simulink subsystem "OFDM_modulator"  (R2022a)
settings: Solver=VariableStepAuto  StartTime=0.0  StopTime=10.0  RelTol=1e-3
values from neighbouring files (symbols this model uses):
  channelNum = fftSize / 2    (= 256)    [initSefdmModel.m]
  frameNum = dataNum + preambleNum    (= 18)    [initSefdmModel.m]
  indiciesWithCP = [issuedSize-cpLength+1:issuedSize, 1:issuedSize]    [initSefdmModel.m]
  paddingN1 = fftSize - (N1+2)    (= 256)    [initSefdmModel.m]
  symbolsPerFrame = bitsPerFrame / bitsPerSymbol    (= 4064)    [initSefdmModel.m]
libraries: dspindex x2, dspxfrm3 x1
settings Model: Creator=lsfan  LastModifiedBy=lsfan

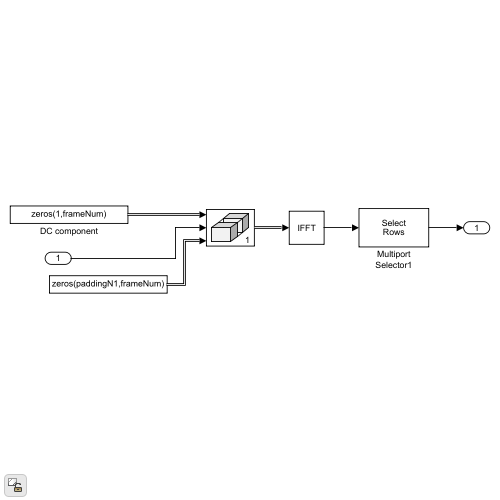
[thumbnail: Simulink's stored preview of the top-level diagram]
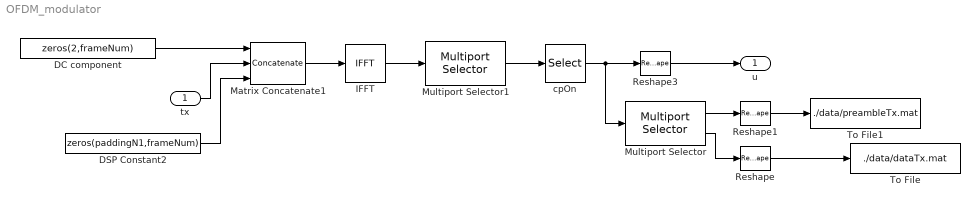
== system OFDM_modulator ==
  tx : Inport
  DC component : Constant  Value=zeros(2,frameNum)  VectorParams1D=off  FramePeriod=Inf
      settings: SamplingMode=Frame based
  DSP Constant2 : Constant  Value=zeros(paddingN1,frameNum)  VectorParams1D=off  FramePeriod=Inf
      settings: SamplingMode=Frame based
  IFFT : dspxfrm3/IFFT  FFTImplementation=Auto  CompMethod=Table lookup  TableOpt=NEW  TableOptActive=Speed  BitRevOrder=off  cs_in=on  Normalize=on  InheritFFTLength=on  FFTLength=64  WrapInput=on  mode=Complex  outSamplingMode=Sample based  roundingMode=Floor  overflowMode=off  firstCoeffDataTypeStr=Inherit: Same word length as input  firstCoeffLastDataTypeStr=Inherit: Same word length as input  outputMin=[]  outputMax=[]
  Matrix Concatenate1 : Concatenate  NumInputs=3  Mode=Multidimensional array
  Multiport Selector : dspindex/Multiport Selector  rowsOrCols=Columns  idxCellArray={[1:preambleNum], [preambleNum+1:frameNum]}  idxErrMode=Clip Index
  Multiport Selector1 : dspindex/Multiport Selector  rowsOrCols=Rows  idxCellArray={channelIssued}  idxErrMode=Clip Index
  Reshape : Reshape
  Reshape1 : Reshape
  Reshape3 : Reshape  OutputDimensions=[channelNum, symbolsPerFrame / channelNum]
  To File : ToFile  Filename=./data/dataTx.mat  SaveFormat=Timeseries
  To File1 : ToFile  Filename=./data/preambleTx.mat  SaveFormat=Timeseries
  cpOn : Selector  NumberOfDimensions=2  InputPortWidth=3  IndexOptions=Index vector (dialog),Select all  Indices=indiciesWithCP,indiciesWithCP  OutputSizes=1,1
  u : Outport
  wires:
  DC component/1 -> Matrix Concatenate1/1
  Multiport Selector1/1 -> cpOn/1
  Multiport Selector/2 -> Reshape/1
  Reshape3/1 -> u/1
  IFFT/1 -> Multiport Selector1/1
  Matrix Concatenate1/1 -> IFFT/1
  DSP Constant2/1 -> Matrix Concatenate1/3
  Multiport Selector/1 -> Reshape1/1
  Reshape1/1 -> To File1/1
  tx/1 -> Matrix Concatenate1/2
  Reshape/1 -> To File/1
  cpOn/1 -> Multiport Selector/1, Reshape3/1
